simulink model "AOE_OBAS"  (R2024b)
settings: Solver=ode4  StartTime=0  StopTime=200  FixedStep=0.01  MaxStep=0.01  RelTol=1e-3
values from neighbouring files (symbols this model uses):
  AOE = Constants_3Body_v2(inputs)    [wecSimInputFile.m]
undefined symbols (not defined in the file or in its folder): body, constraint, DiscIntNeverNeededParam, pto
libraries: WECSim_Lib_Body_Elements x6, simulink x3, WECSim_Lib_Constraints x3, WECSim_Lib_PTOs x3, WECSim_Lib_Frames x1
(part 2 of 2)

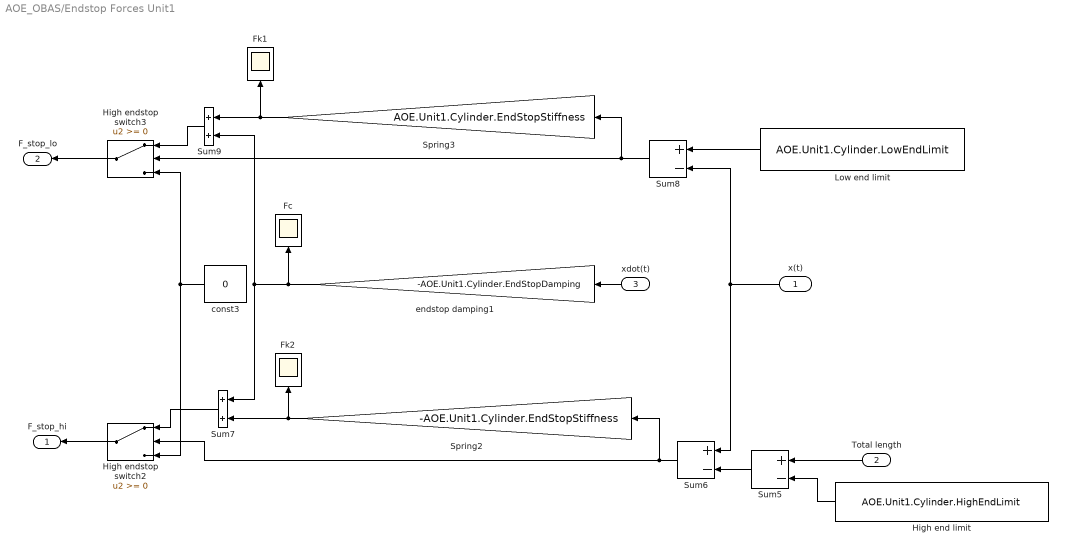
== system AOE_OBAS/Endstop Forces Unit1 ==
  x(t) : Inport
  Total length : Inport  Port=2
  xdot(t) : Inport  Port=3
  Fc : Scope
  Fk1 : Scope
  Fk2 : Scope
  High end limit : Constant  Value=AOE.Unit1.Cylinder.HighEndLimit
  High endstop switch2 : Switch  SaturateOnIntegerOverflow=off  InputSameDT=off
  High endstop switch3 : Switch  SaturateOnIntegerOverflow=off  InputSameDT=off
  Low end limit : Constant  Value=AOE.Unit1.Cylinder.LowEndLimit
  Spring2 : Gain  Gain=-AOE.Unit1.Cylinder.EndStopStiffness
  Spring3 : Gain  Gain=AOE.Unit1.Cylinder.EndStopStiffness
  Sum5 : Sum  Inputs=+-
  Sum6 : Sum  Inputs=+-
  Sum7 : Sum
  Sum8 : Sum  Inputs=+-
  Sum9 : Sum
  const3 : Constant  Value=0
  endstop damping1 : Gain  Gain=-AOE.Unit1.Cylinder.EndStopDamping
  F_stop_hi : Outport
  F_stop_lo : Outport  Port=2
  wires:
  x(t)/1 -> Sum8/2, Sum6/1
  Total length/1 -> Sum5/1
  High end limit/1 -> Sum5/2
  Sum5/1 -> Sum6/2
  Sum6/1 -> High endstop switch2/2, Spring2/1
  Spring2/1 -> Fk2/1, Sum7/2
  const3/1 -> High endstop switch3/3, High endstop switch2/3
  High endstop switch2/1 -> F_stop_hi/1
  xdot(t)/1 -> endstop damping1/1
  endstop damping1/1 -> Sum9/2, Sum7/1, Fc/1
  Sum7/1 -> High endstop switch2/1
  Low end limit/1 -> Sum8/1
  Sum8/1 -> High endstop switch3/2, Spring3/1
  Spring3/1 -> Fk1/1, Sum9/1
  Sum9/1 -> High endstop switch3/1
  High endstop switch3/1 -> F_stop_lo/1

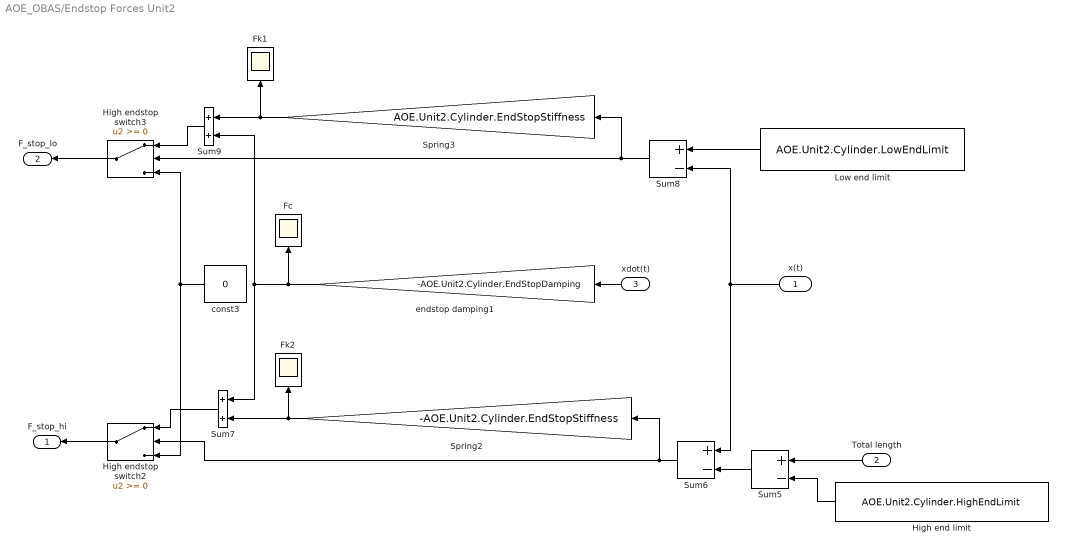
== system AOE_OBAS/Endstop Forces Unit2 ==
  x(t) : Inport
  Total length : Inport  Port=2
  xdot(t) : Inport  Port=3
  Fc : Scope
  Fk1 : Scope
  Fk2 : Scope
  High end limit : Constant  Value=AOE.Unit2.Cylinder.HighEndLimit
  High endstop switch2 : Switch  SaturateOnIntegerOverflow=off  InputSameDT=off
  High endstop switch3 : Switch  SaturateOnIntegerOverflow=off  InputSameDT=off
  Low end limit : Constant  Value=AOE.Unit2.Cylinder.LowEndLimit
  Spring2 : Gain  Gain=-AOE.Unit2.Cylinder.EndStopStiffness
  Spring3 : Gain  Gain=AOE.Unit2.Cylinder.EndStopStiffness
  Sum5 : Sum  Inputs=+-
  Sum6 : Sum  Inputs=+-
  Sum7 : Sum
  Sum8 : Sum  Inputs=+-
  Sum9 : Sum
  const3 : Constant  Value=0
  endstop damping1 : Gain  Gain=-AOE.Unit2.Cylinder.EndStopDamping
  F_stop_hi : Outport
  F_stop_lo : Outport  Port=2
  wires:
  x(t)/1 -> Sum8/2, Sum6/1
  Total length/1 -> Sum5/1
  High end limit/1 -> Sum5/2
  Sum5/1 -> Sum6/2
  Sum6/1 -> High endstop switch2/2, Spring2/1
  Spring2/1 -> Fk2/1, Sum7/2
  const3/1 -> High endstop switch3/3, High endstop switch2/3
  High endstop switch2/1 -> F_stop_hi/1
  xdot(t)/1 -> endstop damping1/1
  endstop damping1/1 -> Sum9/2, Sum7/1, Fc/1
  Sum7/1 -> High endstop switch2/1
  Low end limit/1 -> Sum8/1
  Sum8/1 -> High endstop switch3/2, Spring3/1
  Spring3/1 -> Fk1/1, Sum9/1
  Sum9/1 -> High endstop switch3/1
  High endstop switch3/1 -> F_stop_lo/1

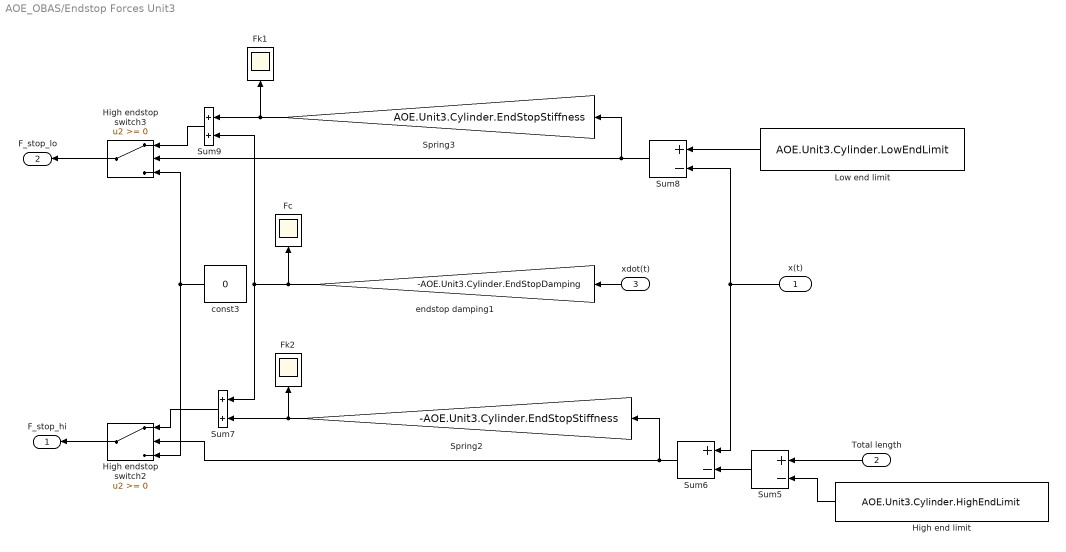
== system AOE_OBAS/Endstop Forces Unit3 ==
  x(t) : Inport
  Total length : Inport  Port=2
  xdot(t) : Inport  Port=3
  Fc : Scope
  Fk1 : Scope
  Fk2 : Scope
  High end limit : Constant  Value=AOE.Unit3.Cylinder.HighEndLimit
  High endstop switch2 : Switch  SaturateOnIntegerOverflow=off  InputSameDT=off
  High endstop switch3 : Switch  SaturateOnIntegerOverflow=off  InputSameDT=off
  Low end limit : Constant  Value=AOE.Unit3.Cylinder.LowEndLimit
  Spring2 : Gain  Gain=-AOE.Unit3.Cylinder.EndStopStiffness
  Spring3 : Gain  Gain=AOE.Unit3.Cylinder.EndStopStiffness
  Sum5 : Sum  Inputs=+-
  Sum6 : Sum  Inputs=+-
  Sum7 : Sum
  Sum8 : Sum  Inputs=+-
  Sum9 : Sum
  const3 : Constant  Value=0
  endstop damping1 : Gain  Gain=-AOE.Unit3.Cylinder.EndStopDamping
  F_stop_hi : Outport
  F_stop_lo : Outport  Port=2
  wires:
  x(t)/1 -> Sum8/2, Sum6/1
  Total length/1 -> Sum5/1
  High end limit/1 -> Sum5/2
  Sum5/1 -> Sum6/2
  Sum6/1 -> High endstop switch2/2, Spring2/1
  Spring2/1 -> Fk2/1, Sum7/2
  const3/1 -> High endstop switch3/3, High endstop switch2/3
  High endstop switch2/1 -> F_stop_hi/1
  xdot(t)/1 -> endstop damping1/1
  endstop damping1/1 -> Sum9/2, Sum7/1, Fc/1
  Sum7/1 -> High endstop switch2/1
  Low end limit/1 -> Sum8/1
  Sum8/1 -> High endstop switch3/2, Spring3/1
  Spring3/1 -> Fk1/1, Sum9/1
  Sum9/1 -> High endstop switch3/1
  High endstop switch3/1 -> F_stop_lo/1

== matlab function AOE_OBAS/Temperature Chamber2 Box Unit1 ==
  data: P input; T output; Rs input; V input; m input
function T = fcn(P,Rs,V,m)

T = P*V/(m*Rs);

== matlab function AOE_OBAS/Pressure Chamber2 Box Unit2 ==
  data: P input; T input; xdot input; x input; Tin1 input; mdot1 input; mdot3 input; L input; A input; D input; Pdot output; Rs input; gma input; Tw input; h input
function Pdot = fcn(P, T,xdot ,x, Tin1, mdot1,mdot3,L,A, D,Rs,gma,Tw,h)

V = A * (x +L);
a = pi*D*(x +L) + 2*A; %heat transfer area

Pdot = (-1*gma*P*(xdot)*A - (gma-1)*h*a*(T-Tw) + gma*Rs*Tin1*mdot1 - gma*Rs*T*mdot3)/V;

== matlab function AOE_OBAS/Temperature Tank Box Unit1 ==
  data: P input; T output; Rs input; V input; m input
function T = fcn(P,Rs,V,m)

T = P*V/(m*Rs);

== matlab function AOE_OBAS/Volume Chamber1 Box Unit1 ==
  data: x input; A input; V output; L input
function V = fcn(x,A,L)
V = A*(-x +L);

== matlab function AOE_OBAS/Volume Chamber2 Box Unit1 ==
  data: x input; A input; V output; L input
function V = fcn(x,A,L)

V = A*(x +L);

== matlab function AOE_OBAS/Revised Valve Model ==
  data: mdotMaxOld input; TimeStep input; PC input; TC input; xdot input; x input; LC input; AC input; DC input; Rs input; gma input; Tw input; hC input; MassFlow output; hT input; aT input; VT input; PT input; TT input; A input; mdotMax output
function [MassFlow, mdotMax]   = fcn(mdotMaxOld, TimeStep, PC, TC,xdot ,x, LC,AC, DC,Rs,gma,Tw,hC, hT, aT, VT, PT, TT, A)

if PC >= PT
    beta = PT/PC;
    
    if beta > 0.999
        beta = 0.999;
    end
    
    if beta > 0.5283
        mdotMax = A*PC*sqrt(abs((2*gma/((gma-1)*Rs*TC))*((beta)^(2/gma) - (beta)^((gma+1)/gma)))); %subsonic
    else
        mdotMax = 0.0404*PC*A/sqrt(TC); %sonic
    end
    
else
    mdotMax = 0;
end

%Calculating Volumes/Areas
VC = AC*(x +LC);
aC = pi*DC*(x +LC) + 2*AC; %heat transfer area

if TimeStep == 0
    MassFlow = 0;
    PdotC = 0;
else
    
    P2 = (TimeStep/(VT+VC))*( (PT*VT/TimeStep) + (PC*VC/TimeStep) - gma*PC*(xdot)*AC - (gma-1)*hC*aC*(TC-Tw) -(gma-1)*hT*aT*(TT-Tw));
    
    MassFlow_Opt = (1/(Rs*TC*gma))*( -(P2 - PC)*VC/TimeStep - gma*PC*(xdot)*AC - (gma-1)*hC*aC*(TC-Tw) );
    
    MassFlow = MassFlow_Opt*0.99;
    
    PdotC = (-1*gma*PC*(xdot)*AC - (gma-1)*hC*aC*(TC-Tw) - gma*Rs*TC*MassFlow )/VC;
end

if MassFlow < 0
    MassFlow = 0;
end

if MassFlow > mdotMax
    if mdotMaxOld > mdotMax
        if MassFlow > mdotMaxOld
            MassFlow = mdotMaxOld;
        end
        mdotMax = mdotMaxOld;
    else
        MassFlow = mdotMax;
    end
end

== matlab function AOE_OBAS/Revised Valve Tank Outlet Unit1 ==
  data: mdotMaxOld input; TimeStep input; PT input; TT input; Rs input; gma input; Tw input; hT input; VT input; aT input; TC input; mDotIn input; A input; VP input; aP input; MassFlow output; mdotMax output; hP input; PP input; TP input
function [MassFlow, mdotMax]   = fcn(mdotMaxOld, TimeStep, PT, TT ,Rs,gma,Tw,hT, VT, aT, TC, mDotIn, A, VP, aP, hP, PP, TP)

%Determine Maximum Mass Flow Rate

%A is orifice area

if PT >= PP
    beta = PP/PT;
    
    %This prevents instabilities as Beta approaches 1
    if beta > 0.999
        beta = 0.999;
    end
    
    if beta > 0.5283
        mdotMax = A*PT*sqrt(abs((2*gma/((gma-1)*Rs*TT))*((beta)^(2/gma) - (beta)^((gma+1)/gma)))); %subsonic
    else
        mdotMax = 0.0404*PT*A/sqrt(TT); %sonic
    end
    
else
    mdotMax = 0;
    beta = 0;
end

if TimeStep == 0
    MassFlow = 0;
else
    %Determining what the pressure needs to be in the following time step
    P2 = (TimeStep/(VP + VT))*( (PP*VP/TimeStep) + (PT*VT/TimeStep) - (gma - 1)*hP*aP*(TP - Tw) - (gma - 1)*hT*aT*(TT - Tw) + gma*Rs*TC*mDotIn);
    
    MassFlow_Opt = (1/(Rs*TT*gma))*( -(P2 - PT)*VT/TimeStep - (gma-1)*hT*aT*(TT-Tw) + gma*Rs*TC*mDotIn);
    %MassFlow_Opt2 = (1/(Rs*TT*gma))*( (P2 - PC1)*VC/TimeStep + gma*PC1*(-xDot)*AC + (gma - 1)*hC*aC*(TC1 - Tw) )

    MassFlow = MassFlow_Opt*0.99;
end

if MassFlow < 0
    MassFlow = 0;
end

if MassFlow > mdotMax
    if mdotMaxOld > mdotMax
        if MassFlow > mdotMaxOld
            MassFlow = mdotMaxOld;
        end
        mdotMax = mdotMaxOld;
    else
        MassFlow = mdotMax;
    end
end
    
end

== matlab function AOE_OBAS/Revised Valve Model Inlet Unit1 ==
  data: mdotMaxOld input; TimeStep input; PC1 input; TC1 input; xdot input; x input; LC input; AC input; DC input; Rs input; gma input; Tw input; hC input; Tamb input; A input; MassFlow output; Pamb input; mdotMax output
function [MassFlow, mdotMax]   = fcn(mdotMaxOld, TimeStep, PC1, TC1,xdot ,x, LC,AC, DC,Rs,gma,Tw,hC, Tamb, A, Pamb)

if Pamb >= PC1
    beta = PC1/Pamb;
    
    if beta > 0.999
        beta = 0.999;
    end
    
    if beta > 0.5283
        mdotMax = A*Pamb*sqrt(abs((2*gma/((gma-1)*Rs*Tamb))*((beta)^(2/gma) - (beta)^((gma+1)/gma)))); %subsonic
    else
        mdotMax = 0.0404*Pamb*A/sqrt(Tamb); %sonic
    end
    
else
    mdotMax = 0;
end

if TimeStep == 0
    MassFlow = 0;
else
    %Calculating Volumes/Areas
    VC = AC*(-x +LC);
    aC = pi*DC*(-x +LC) + 2*AC; %heat transfer area
    
    %Determining what the pressure needs to be in the following time step
    P2 = Pamb;
    
    MassFlow_Opt = (1/(Rs*Tamb*gma))*( (P2 - PC1)*VC/TimeStep + gma*PC1*(-xdot)*AC + (gma-1)*hC*aC*(TC1-Tw) );
    MassFlow = MassFlow_Opt*0.99;

end

if MassFlow < 0
    MassFlow = 0;
end

if MassFlow > mdotMax
    if mdotMaxOld > mdotMax
        if MassFlow > mdotMaxOld
            MassFlow = mdotMaxOld;
        end
        mdotMax = mdotMaxOld;
    else
        MassFlow = mdotMax;
    end
end

== matlab function AOE_OBAS/Revised Valve Model Chamber1Chamber2 Unit1 ==
  data: mdotMaxOld input; TimeStep input; xdot input; x input; PC1 input; TC1 input; LC input; AC input; DC input; Rs input; gma input; Tw input; hC input; MassFlow output; PC2 input; TC2 input; A input; mdotMax output
function [MassFlow, mdotMax]   = fcn(mdotMaxOld, TimeStep, xdot ,x,PC1, TC1, LC,AC, DC,Rs,gma,Tw,hC, PC2, TC2, A)

if PC1 >= PC2
    beta = PC2/PC1;
    
    if beta > 0.999
        beta = 0.999;
    end
    
    if beta > 0.5283
        mdotMax = A*PC1*sqrt(abs((2*gma/((gma-1)*Rs*TC1))*((beta)^(2/gma) - (beta)^((gma+1)/gma)))); %subsonic
    else
        mdotMax = 0.0404*PC1*A/sqrt(TC1); %sonic
    end
    
else
    mdotMax = 0;
end

if TimeStep == 0
    MassFlow = 0;
else
    %Calculating Volumes/Areas
    VC1 = AC*(-x +LC);
    aC1 = pi*DC*(-x +LC) + 2*AC; %heat transfer area
    
    VC2 = AC*(x +LC);
    aC2 = pi*DC*(x +LC) + 2*AC; %heat transfer area
    
    %Determining what the pressure needs to be in the following time step
    P2 = (TimeStep/(VC2+VC1))*( (PC2*VC2/TimeStep) + (PC1*VC1/TimeStep) - gma*PC1*(-xdot)*AC - (gma-1)*hC*aC1*(TC1-Tw) - gma*PC2*xdot*AC - (gma-1)*hC*aC2*(TC2-Tw));
    
    MassFlow_Opt = (1/(Rs*TC1*gma))*( -(P2 - PC1)*VC1/TimeStep - gma*PC1*(-xdot)*AC - (gma-1)*hC*aC1*(TC1-Tw) );
    MassFlow = MassFlow_Opt*0.99;

end

if MassFlow < 0
    MassFlow = 0;
end

if MassFlow > mdotMax
    if mdotMaxOld > mdotMax
        if MassFlow > mdotMaxOld
            MassFlow = mdotMaxOld;
        end
        mdotMax = mdotMaxOld;
    else
        MassFlow = mdotMax;
    end
end

== matlab function AOE_OBAS/Pressure Tank Box Unit2 ==
  data: T input; Tin input; mdot1 input; mdot2 input; Rs input; gma input; h input; a input; V input; Tw input; Pdot output
function Pdot  = fcn(T, Tin, mdot1,mdot2,Rs,gma,h, a, V,Tw)

Pdot = (-(gma-1)*h*a*(T-Tw) + gma*Rs*Tin*mdot1 - gma*Rs*T*mdot2)/V;

== matlab function AOE_OBAS/Revised Valve Model Chamber1Chamber2 Unit2 ==
  data: mdotMaxOld input; TimeStep input; xdot input; x input; PC1 input; TC1 input; LC input; AC input; DC input; Rs input; gma input; Tw input; hC input; MassFlow output; PC2 input; TC2 input; A input; mdotMax output
function [MassFlow, mdotMax]   = fcn(mdotMaxOld, TimeStep, xdot ,x,PC1, TC1, LC,AC, DC,Rs,gma,Tw,hC, PC2, TC2, A)

if PC1 >= PC2
    beta = PC2/PC1;
    
    if beta > 0.999
        beta = 0.999;
    end
    
    if beta > 0.5283
        mdotMax = A*PC1*sqrt(abs((2*gma/((gma-1)*Rs*TC1))*((beta)^(2/gma) - (beta)^((gma+1)/gma)))); %subsonic
    else
        mdotMax = 0.0404*PC1*A/sqrt(TC1); %sonic
    end
    
else
    mdotMax = 0;
end

if TimeStep == 0
    MassFlow = 0;
else
    %Calculating Volumes/Areas
    VC1 = AC*(-x +LC);
    aC1 = pi*DC*(-x +LC) + 2*AC; %heat transfer area
    
    VC2 = AC*(x +LC);
    aC2 = pi*DC*(x +LC) + 2*AC; %heat transfer area
    
    %Determining what the pressure needs to be in the following time step
    P2 = (TimeStep/(VC2+VC1))*( (PC2*VC2/TimeStep) + (PC1*VC1/TimeStep) - gma*PC1*(-xdot)*AC - (gma-1)*hC*aC1*(TC1-Tw) - gma*PC2*xdot*AC - (gma-1)*hC*aC2*(TC2-Tw));
    
    MassFlow_Opt = (1/(Rs*TC1*gma))*( -(P2 - PC1)*VC1/TimeStep - gma*PC1*(-xdot)*AC - (gma-1)*hC*aC1*(TC1-Tw) );
    MassFlow = MassFlow_Opt*0.99;

end

if MassFlow < 0
    MassFlow = 0;
end

if MassFlow > mdotMax
    if mdotMaxOld > mdotMax
        if MassFlow > mdotMaxOld
            MassFlow = mdotMaxOld;
        end
        mdotMax = mdotMaxOld;
    else
        MassFlow = mdotMax;
    end
end

== matlab function AOE_OBAS/Revised Valve Tank Outlet Unit2 ==
  data: mdotMaxOld input; TimeStep input; PT input; TT input; Rs input; gma input; Tw input; hT input; VT input; aT input; TC input; mDotIn input; A input; VP input; aP input; MassFlow output; hP input; mdotMax output; PP input; TP input
function [MassFlow, mdotMax]   = fcn(mdotMaxOld, TimeStep, PT, TT ,Rs,gma,Tw,hT, VT, aT, TC, mDotIn, A, VP, aP, hP, PP, TP)

%Determine Maximum Mass Flow Rate

%A is orifice area

if PT >= PP
    beta = PP/PT;
    
    %This prevents instabilities as Beta approaches 1
    if beta > 0.999
        beta = 0.999;
    end
    
    if beta > 0.5283
        mdotMax = A*PT*sqrt(abs((2*gma/((gma-1)*Rs*TT))*((beta)^(2/gma) - (beta)^((gma+1)/gma)))); %subsonic
    else
        mdotMax = 0.0404*PT*A/sqrt(TT); %sonic
    end
    
else
    mdotMax = 0;
    beta = 0;
end

if TimeStep == 0
    MassFlow = 0;
else
    %Determining what the pressure needs to be in the following time step
    P2 = (TimeStep/(VP + VT))*( (PP*VP/TimeStep) + (PT*VT/TimeStep) - (gma - 1)*hP*aP*(TP - Tw) - (gma - 1)*hT*aT*(TT - Tw) + gma*Rs*TC*mDotIn);
    
    MassFlow_Opt = (1/(Rs*TT*gma))*( -(P2 - PT)*VT/TimeStep - (gma-1)*hT*aT*(TT-Tw) + gma*Rs*TC*mDotIn);
    %MassFlow_Opt2 = (1/(Rs*TT*gma))*( (P2 - PC1)*VC/TimeStep + gma*PC1*(-xDot)*AC + (gma - 1)*hC*aC*(TC1 - Tw) )

    MassFlow = MassFlow_Opt*0.99;
end

if MassFlow < 0
    MassFlow = 0;
end

if MassFlow > mdotMax
    if mdotMaxOld > mdotMax
        if MassFlow > mdotMaxOld
            MassFlow = mdotMaxOld;
        end
        mdotMax = mdotMaxOld;
    else
        MassFlow = mdotMax;
    end
end
    
end

== matlab function AOE_OBAS/Pressure Chamber1 Box Unit1 ==
  data: P input; T input; xdot input; x input; Tin1 input; mdot1 input; mdot3 input; L input; A input; D input; Rs input; gma input; Tw input; h input; Pdot output
function Pdot = fcn(P, T,xdot ,x, Tin1, mdot1,mdot3,L,A, D,Rs,gma,Tw,h)

V = A*(-x +L);
a = pi*D*(-x +L) + 2*A; %heat transfer area

Pdot = (-1*gma*P*(-xdot)*A - (gma-1)*h*a*(T-Tw) + gma*Rs*Tin1*mdot1 - gma*Rs*T*mdot3)/V;

== matlab function AOE_OBAS/Pressure Tank Box Unit1 ==
  data: T input; Tin input; mdot1 input; mdot2 input; Rs input; gma input; h input; a input; V input; Tw input; Pdot output
function Pdot  = fcn(T, Tin, mdot1,mdot2,Rs,gma,h, a, V,Tw)

Pdot = (-(gma-1)*h*a*(T-Tw) + gma*Rs*Tin*mdot1 - gma*Rs*T*mdot2)/V;

== matlab function AOE_OBAS/Revised Valve Model Piston Outlet Unit2 ==
  data: mdotMaxOld input; TimeStep input; PC input; TC input; xdot input; x input; LC input; AC input; DC input; Rs input; gma input; Tw input; hC input; MassFlow output; hT input; aT input; VT input; PT input; TT input; A input; mdotMax output
function [MassFlow, mdotMax]   = fcn(mdotMaxOld, TimeStep, PC, TC,xdot ,x, LC,AC, DC,Rs,gma,Tw,hC, hT, aT, VT, PT, TT, A)

if PC >= PT
    beta = PT/PC;
    
    if beta > 0.999
        beta = 0.999;
    end
    
    if beta > 0.5283
        mdotMax = A*PC*sqrt(abs((2*gma/((gma-1)*Rs*TC))*((beta)^(2/gma) - (beta)^((gma+1)/gma)))); %subsonic
    else
        mdotMax = 0.0404*PC*A/sqrt(TC); %sonic
    end
    
else
    mdotMax = 0;
end

%Calculating Volumes/Areas
VC = AC*(x +LC);
aC = pi*DC*(x +LC) + 2*AC; %heat transfer area

if TimeStep == 0
    MassFlow = 0;
else

    P2 = (TimeStep/(VT+VC))*( (PT*VT/TimeStep) + (PC*VC/TimeStep) - gma*PC*(xdot)*AC - (gma-1)*hC*aC*(TC-Tw) -(gma-1)*hT*aT*(TT-Tw));
    
    MassFlow_Opt = (1/(Rs*TC*gma))*( -(P2 - PC)*VC/TimeStep - gma*PC*(xdot)*AC - (gma-1)*hC*aC*(TC-Tw) );
    
    MassFlow = MassFlow_Opt*0.99;
    
    PdotC = (-1*gma*PC*(xdot)*AC - (gma-1)*hC*aC*(TC-Tw) - gma*Rs*TC*MassFlow )/VC;
end

if MassFlow < 0
    MassFlow = 0;
end

if MassFlow > mdotMax
    if mdotMaxOld > mdotMax
        if MassFlow > mdotMaxOld
            MassFlow = mdotMaxOld;
        end
        mdotMax = mdotMaxOld;
    else
        MassFlow = mdotMax;
    end
end

== matlab function AOE_OBAS/Determining Useful Energy ==
  data: T input; P input; mDot input; Density input; Cp input; Rs input; Tamb input; Pamb input; Exergy output; Power output
function [Exergy, Power]   = fcn(T, P, mDot, Density, Cp, Rs, Tamb, Pamb)
    
%Determining Flow Exergy
Flow_Exergy = Cp*Tamb*( (T/Tamb) - 1 - log(T/Tamb) ) + Rs*Tamb*log(P/Pamb);

Exergy = Flow_Exergy*mDot; %This has the units of Watts

%Determining Energy of Output
Power = mDot*(P - Pamb)/Density;

end

== matlab function AOE_OBAS/Temperature Chamber1 Box Unit2 ==
  data: P input; T output; Rs input; V input; m input
function T = fcn(P,Rs,V,m)
T = P*V/(m*Rs);

== matlab function AOE_OBAS/Temperature Chamber2 Box Unit2 ==
  data: P input; T output; Rs input; V input; m input
function T = fcn(P,Rs,V,m)

T = P*V/(m*Rs);

== matlab function AOE_OBAS/Temperature Tank Box Unit2 ==
  data: P input; T output; Rs input; V input; m input
function T = fcn(P,Rs,V,m)

T = P*V/(m*Rs);

== matlab function AOE_OBAS/Volume Chamber1 Box Unit2 ==
  data: x input; A input; V output; L input
function V = fcn(x,A,L)
V = A*(-x +L);

== matlab function AOE_OBAS/Volume Chamber2 Box Unit2 ==
  data: x input; A input; V output; L input
function V = fcn(x,A,L)

V = A*(x +L);

== matlab function AOE_OBAS/Pressure Chamber1 Box Unit3 ==
  data: P input; T input; xdot input; x input; Tin1 input; mdot1 input; mdot3 input; L input; A input; D input; Rs input; gma input; Tw input; h input; Pdot output
function Pdot = fcn(P, T,xdot ,x, Tin1, mdot1,mdot3,L,A, D,Rs,gma,Tw,h)

V = A*(-x +L);
a = pi*D*(-x +L) + 2*A; %heat transfer area

Pdot = (-1*gma*P*(-xdot)*A - (gma-1)*h*a*(T-Tw) + gma*Rs*Tin1*mdot1 - gma*Rs*T*mdot3)/V;

== matlab function AOE_OBAS/Pressure Chamber2 Box Unit3 ==
  data: P input; T input; xdot input; x input; Tin1 input; mdot1 input; mdot3 input; L input; A input; D input; Pdot output; Rs input; gma input; Tw input; h input
function Pdot = fcn(P, T,xdot ,x, Tin1, mdot1,mdot3,L,A, D,Rs,gma,Tw,h)

V = A * (x +L);
a = pi*D*(x +L) + 2*A; %heat transfer area

Pdot = (-1*gma*P*(xdot)*A - (gma-1)*h*a*(T-Tw) + gma*Rs*Tin1*mdot1 - gma*Rs*T*mdot3)/V;

== matlab function AOE_OBAS/Pressure Tank Box Unit3 ==
  data: T input; Tin input; mdot1 input; mdot2 input; Rs input; gma input; h input; a input; V input; Tw input; Pdot output
function Pdot  = fcn(T, Tin, mdot1,mdot2,Rs,gma,h, a, V,Tw)

Pdot = (-(gma-1)*h*a*(T-Tw) + gma*Rs*Tin*mdot1 - gma*Rs*T*mdot2)/V;

== matlab function AOE_OBAS/Revised Valve Model Chamber1Chamber2 Unit3 ==
  data: mdotMaxOld input; TimeStep input; xdot input; x input; PC1 input; TC1 input; LC input; AC input; DC input; Rs input; gma input; Tw input; hC input; MassFlow output; PC2 input; TC2 input; A input; mdotMax output
function [MassFlow, mdotMax]   = fcn(mdotMaxOld, TimeStep, xdot ,x,PC1, TC1, LC,AC, DC,Rs,gma,Tw,hC, PC2, TC2, A)

if PC1 >= PC2
    beta = PC2/PC1;
    
    if beta > 0.999
        beta = 0.999;
    end
    
    if beta > 0.5283
        mdotMax = A*PC1*sqrt(abs((2*gma/((gma-1)*Rs*TC1))*((beta)^(2/gma) - (beta)^((gma+1)/gma)))); %subsonic
    else
        mdotMax = 0.0404*PC1*A/sqrt(TC1); %sonic
    end
    
else
    mdotMax = 0;
end

if TimeStep == 0
    MassFlow = 0;
else
    %Calculating Volumes/Areas
    VC1 = AC*(-x +LC);
    aC1 = pi*DC*(-x +LC) + 2*AC; %heat transfer area
    
    VC2 = AC*(x +LC);
    aC2 = pi*DC*(x +LC) + 2*AC; %heat transfer area
    
    %Determining what the pressure needs to be in the following time step
    P2 = (TimeStep/(VC2+VC1))*( (PC2*VC2/TimeStep) + (PC1*VC1/TimeStep) - gma*PC1*(-xdot)*AC - (gma-1)*hC*aC1*(TC1-Tw) - gma*PC2*xdot*AC - (gma-1)*hC*aC2*(TC2-Tw));
    
    MassFlow_Opt = (1/(Rs*TC1*gma))*( -(P2 - PC1)*VC1/TimeStep - gma*PC1*(-xdot)*AC - (gma-1)*hC*aC1*(TC1-Tw) );
    MassFlow = MassFlow_Opt*0.99;

end

if MassFlow < 0
    MassFlow = 0;
end

if MassFlow > mdotMax
    if mdotMaxOld > mdotMax
        if MassFlow > mdotMaxOld
            MassFlow = mdotMaxOld;
        end
        mdotMax = mdotMaxOld;
    else
        MassFlow = mdotMax;
    end
end

== matlab function AOE_OBAS/Determining Useful Energy1 ==
  data: T input; P input; mDot input; Density input; Cp input; Rs input; Tamb input; Pamb input; Exergy output; Power output
function [Exergy, Power]   = fcn(T, P, mDot, Density, Cp, Rs, Tamb, Pamb)
    
%Determining Flow Exergy
Flow_Exergy = Cp*Tamb*( (T/Tamb) - 1 - log(T/Tamb) ) + Rs*Tamb*log(P/Pamb);

Exergy = Flow_Exergy*mDot; %This has the units of Watts

%Determining Energy of Output
Power = mDot*(P - Pamb)/Density;

end

== matlab function AOE_OBAS/Revised Valve Model Piston Outlet Unit3 ==
  data: mdotMaxOld input; TimeStep input; PC input; TC input; xdot input; x input; LC input; AC input; DC input; Rs input; gma input; Tw input; hC input; MassFlow output; hT input; aT input; VT input; PT input; TT input; A input; mdotMax output
function [MassFlow, mdotMax]   = fcn(mdotMaxOld, TimeStep, PC, TC,xdot ,x, LC,AC, DC,Rs,gma,Tw,hC, hT, aT, VT, PT, TT, A)

if PC >= PT
    beta = PT/PC;
    
    if beta > 0.999
        beta = 0.999;
    end
    
    if beta > 0.5283
        mdotMax = A*PC*sqrt(abs((2*gma/((gma-1)*Rs*TC))*((beta)^(2/gma) - (beta)^((gma+1)/gma)))); %subsonic
    else
        mdotMax = 0.0404*PC*A/sqrt(TC); %sonic
    end
    
else
    mdotMax = 0;
end

%Calculating Volumes/Areas
VC = AC*(x +LC);
aC = pi*DC*(x +LC) + 2*AC; %heat transfer area

if TimeStep == 0
    MassFlow = 0;
else
    P2 = (TimeStep/(VT+VC))*( (PT*VT/TimeStep) + (PC*VC/TimeStep) - gma*PC*(xdot)*AC - (gma-1)*hC*aC*(TC-Tw) -(gma-1)*hT*aT*(TT-Tw));
    
    MassFlow_Opt = (1/(Rs*TC*gma))*( -(P2 - PC)*VC/TimeStep - gma*PC*(xdot)*AC - (gma-1)*hC*aC*(TC-Tw) );
    
    MassFlow = MassFlow_Opt*0.99;
    
    PdotC = (-1*gma*PC*(xdot)*AC - (gma-1)*hC*aC*(TC-Tw) - gma*Rs*TC*MassFlow )/VC;
end

if MassFlow < 0
    MassFlow = 0;
end

if MassFlow > mdotMax
    if mdotMaxOld > mdotMax
        if MassFlow > mdotMaxOld
            MassFlow = mdotMaxOld;
        end
        mdotMax = mdotMaxOld;
    else
        MassFlow = mdotMax;
    end
end

== matlab function AOE_OBAS/Revised Valve Tank Outlet2 ==
  data: mdotMaxOld input; TimeStep input; PT input; TT input; Rs input; gma input; Tw input; hT input; VT input; aT input; MassFlow output; Pcrack input; TC input; mDotIn input; A input; mdotMax output
function [MassFlow, mdotMax]   = fcn(mdotMaxOld, TimeStep, PT, TT ,Rs,gma,Tw,hT, VT, aT, Pcrack, TC, mDotIn, A)

%Determine Maximum Mass Flow Rate

%A is orifice area

if PT >= Pcrack
    beta = Pcrack/PT;
    
    %This prevents instabilities as Beta approaches 1
    if beta > 0.999
        beta = 0.999;
    end
    
    if beta > 0.5283
        mdotMax = A*PT*sqrt(abs((2*gma/((gma-1)*Rs*TT))*((beta)^(2/gma) - (beta)^((gma+1)/gma)))); %subsonic
    else
        mdotMax = 0.0404*PT*A/sqrt(TT); %sonic
    end
    
else
    mdotMax = 0;
    beta = 0;
end

if TimeStep == 0
    MassFlow = 0;
else
    %Determining what the pressure needs to be in the following time step
    P2 = Pcrack;
    
    MassFlow_Opt = (1/(Rs*TT*gma))*( -(P2 - PT)*VT/TimeStep - (gma-1)*hT*aT*(TT-Tw) + gma*Rs*TC*mDotIn);
    
    MassFlow = MassFlow_Opt*0.99;
end

if MassFlow < 0
    MassFlow = 0;
end

if MassFlow > mdotMax
    if mdotMaxOld > mdotMax
        if MassFlow > mdotMaxOld
            MassFlow = mdotMaxOld;
        end
        mdotMax = mdotMaxOld;
    else
        MassFlow = mdotMax;
    end
end
    
end

== matlab function AOE_OBAS/Temperature Chamber1 Box Unit3 ==
  data: P input; T output; Rs input; V input; m input
function T = fcn(P,Rs,V,m)
T = P*V/(m*Rs);

== matlab function AOE_OBAS/Temperature Chamber2 Box Unit3 ==
  data: P input; T output; Rs input; V input; m input
function T = fcn(P,Rs,V,m)

T = P*V/(m*Rs);

== matlab function AOE_OBAS/Temperature Tank Box Unit3 ==
  data: P input; T output; Rs input; V input; m input
function T = fcn(P,Rs,V,m)

T = P*V/(m*Rs);

== matlab function AOE_OBAS/Pressure Chamber1 Box Unit2 ==
  data: P input; T input; xdot input; x input; Tin1 input; mdot1 input; mdot3 input; L input; A input; D input; Rs input; gma input; Tw input; h input; Pdot output
function Pdot = fcn(P, T,xdot ,x, Tin1, mdot1,mdot3,L,A, D,Rs,gma,Tw,h)

V = A*(-x +L);
a = pi*D*(-x +L) + 2*A; %heat transfer area

Pdot = (-1*gma*P*(-xdot)*A - (gma-1)*h*a*(T-Tw) + gma*Rs*Tin1*mdot1 - gma*Rs*T*mdot3)/V;

== matlab function AOE_OBAS/Volume Chamber1 Box Unit3 ==
  data: x input; A input; V output; L input
function V = fcn(x,A,L)
V = A*(-x +L);

== matlab function AOE_OBAS/Volume Chamber2 Box Unit3 ==
  data: x input; A input; V output; L input
function V = fcn(x,A,L)

V = A*(x +L);

== matlab function AOE_OBAS/Determining Useful Energy2 ==
  data: T input; P input; mDot input; Density input; Cp input; Rs input; Tamb input; Pamb input; Exergy output; Power output
function [Exergy, Power]   = fcn(T, P, mDot, Density, Cp, Rs, Tamb, Pamb)
    
%Determining Flow Exergy
Flow_Exergy = Cp*Tamb*( (T/Tamb) - 1 - log(T/Tamb) ) + Rs*Tamb*log(P/Pamb);

Exergy = Flow_Exergy*mDot; %This has the units of Watts

%Determining Energy of Output
Power = mDot*(P - Pamb)/Density;

end

== matlab function AOE_OBAS/Pipe Unit1 to Unit1 ==
  data: T input; Tin input; mdot1 input; mdot2 input; Rs input; gma input; h input; a input; V input; Tw input; Pdot output
function Pdot  = fcn(T, Tin, mdot1,mdot2,Rs,gma,h, a, V, Tw)

Pdot = (-(gma-1)*h*a*(T-Tw) + gma*Rs*Tin*mdot1 - gma*Rs*T*mdot2)/V;

== matlab function AOE_OBAS/Revised Valve Pipe Outlet Unit2 ==
  data: mdotMaxOld input; TimeStep input; PP input; TP input; Rs input; gma input; Tw input; hP input; VP input; aP input; TT input; mDotIn input; A input; AC input; x input; MassFlow output; xDot input; mdotMax output; LC input; hC input; DC input; PC1 input; TC1 input
function [MassFlow, mdotMax]   = fcn(mdotMaxOld, TimeStep, PP, TP ,Rs,gma,Tw,hP, VP, aP, TT, mDotIn, A, AC, x, xDot, LC, hC, DC, PC1, TC1)

%Determine Maximum Mass Flow Rate

%A is orifice area

if PP >= PC1
    beta = PC1/PP;
    
    %This prevents instabilities as Beta approaches 1
    if beta > 0.999
        beta = 0.999;
    end
    
    if beta > 0.5283
        mdotMax = A*PP*sqrt(abs((2*gma/((gma-1)*Rs*TP))*((beta)^(2/gma) - (beta)^((gma+1)/gma)))); %subsonic
    else
        mdotMax = 0.0404*PP*A/sqrt(TP); %sonic
    end
    
else
    mdotMax = 0;
    beta = 0;
end

if TimeStep == 0
    MassFlow = 0;
else
    %Determining what the pressure needs to be in the following time step
    VC = AC*(-x +LC);
    aC = pi*DC*(-x +LC) + 2*AC; %heat transfer area

    P2 = (TimeStep/(VC + VP))*( (PC1*VC/TimeStep) + (PP*VP/TimeStep) - gma*PC1*(-xDot)*AC - (gma - 1)*hC*aC*(TC1 - Tw) - (gma - 1)*hP*aP*(TP - Tw) + gma*Rs*TT*mDotIn);
    
    MassFlow_Opt = (1/(Rs*TP*gma))*( -(P2 - PP)*VP/TimeStep - (gma-1)*hP*aP*(TP-Tw) + gma*Rs*TT*mDotIn);
    %MassFlow_Opt2 = (1/(Rs*TT*gma))*( (P2 - PC1)*VC/TimeStep + gma*PC1*(-xDot)*AC + (gma - 1)*hC*aC*(TC1 - Tw) )

    MassFlow = MassFlow_Opt*0.99;
end

if MassFlow < 0
    MassFlow = 0;
end

if MassFlow > mdotMax
    if mdotMaxOld > mdotMax
        if MassFlow > mdotMaxOld
            MassFlow = mdotMaxOld;
        end
        mdotMax = mdotMaxOld;
    else
        MassFlow = mdotMax;
    end
end
    
end

== matlab function AOE_OBAS/Temperature Pipe Unit1 to Unit1 ==
  data: P input; T output; Rs input; V input; m input
function T = fcn(P,Rs,V,m)

T = P*V/(m*Rs);

== matlab function AOE_OBAS/Pipe Unit1 to Unit2 ==
  data: T input; Tin input; mdot1 input; mdot2 input; Rs input; gma input; h input; a input; V input; Tw input; Pdot output
function Pdot  = fcn(T, Tin, mdot1,mdot2,Rs,gma,h, a, V, Tw)

Pdot = (-(gma-1)*h*a*(T-Tw) + gma*Rs*Tin*mdot1 - gma*Rs*T*mdot2)/V;

== matlab function AOE_OBAS/Revised Valve Pipe Outlet Unit1 ==
  data: mdotMaxOld input; TimeStep input; PP input; TP input; Rs input; gma input; Tw input; hP input; VP input; aP input; TT input; mDotIn input; A input; AC input; x input; MassFlow output; xDot input; mdotMax output; LC input; hC input; DC input; PC1 input; TC1 input
function [MassFlow, mdotMax]   = fcn(mdotMaxOld, TimeStep, PP, TP ,Rs,gma,Tw,hP, VP, aP, TT, mDotIn, A, AC, x, xDot, LC, hC, DC, PC1, TC1)

%Determine Maximum Mass Flow Rate

%A is orifice area

if PP >= PC1
    beta = PC1/PP;
    
    %This prevents instabilities as Beta approaches 1
    if beta > 0.999
        beta = 0.999;
    end
    
    if beta > 0.5283
        mdotMax = A*PP*sqrt(abs((2*gma/((gma-1)*Rs*TP))*((beta)^(2/gma) - (beta)^((gma+1)/gma)))); %subsonic
    else
        mdotMax = 0.0404*PP*A/sqrt(TP); %sonic
    end
    
else
    mdotMax = 0;
    beta = 0;
end

if TimeStep == 0
    MassFlow = 0;
else
    %Determining what the pressure needs to be in the following time step
    VC = AC*(-x +LC);
    aC = pi*DC*(-x +LC) + 2*AC; %heat transfer area

    P2 = (TimeStep/(VC + VP))*( (PC1*VC/TimeStep) + (PP*VP/TimeStep) - gma*PC1*(-xDot)*AC - (gma - 1)*hC*aC*(TC1 - Tw) - (gma - 1)*hP*aP*(TP - Tw) + gma*Rs*TT*mDotIn);
    
    MassFlow_Opt = (1/(Rs*TP*gma))*( -(P2 - PP)*VP/TimeStep - (gma-1)*hP*aP*(TP-Tw) + gma*Rs*TT*mDotIn);
    %MassFlow_Opt2 = (1/(Rs*TT*gma))*( (P2 - PC1)*VC/TimeStep + gma*PC1*(-xDot)*AC + (gma - 1)*hC*aC*(TC1 - Tw) )

    MassFlow = MassFlow_Opt*0.99;
end

if MassFlow < 0
    MassFlow = 0;
end

if MassFlow > mdotMax
    if mdotMaxOld > mdotMax
        if MassFlow > mdotMaxOld
            MassFlow = mdotMaxOld;
        end
        mdotMax = mdotMaxOld;
    else
        MassFlow = mdotMax;
    end
end
    
end

== matlab function AOE_OBAS/Temperature Pipe Unit1 to Unit2 ==
  data: P input; T output; Rs input; V input; m input
function T = fcn(P,Rs,V,m)

T = P*V/(m*Rs);

== matlab function AOE_OBAS/Temperature Chamber1 Box Unit1 ==
  data: P input; T output; Rs input; V input; m input
function T = fcn(P,Rs,V,m)
T = P*V/(m*Rs);

== matlab function AOE_OBAS/Pressure Chamber2 Box Unit1 ==
  data: P input; T input; xdot input; x input; Tin1 input; mdot1 input; mdot3 input; L input; A input; D input; Pdot output; Rs input; gma input; Tw input; h input
function Pdot = fcn(P, T,xdot ,x, Tin1, mdot1,mdot3,L,A, D,Rs,gma,Tw,h)

V = A * (x +L);
a = pi*D*(x +L) + 2*A; %heat transfer area

Pdot = (-1*gma*P*(xdot)*A - (gma-1)*h*a*(T-Tw) + gma*Rs*Tin1*mdot1 - gma*Rs*T*mdot3)/V;
